simulink model "Scenario_1_fuzzy_tuning"  (R2025b)
settings: Solver=VariableStepAuto  StartTime=0.0  StopTime=10.0  RelTol=1e-3
model workspace (MAT data in the model file):
  Ke = 1
  a = 1
  a1 = 0.1
libraries: fuzblock x2, slpidlib x1
settings Model: Creator=danai  LastModifiedBy=danai

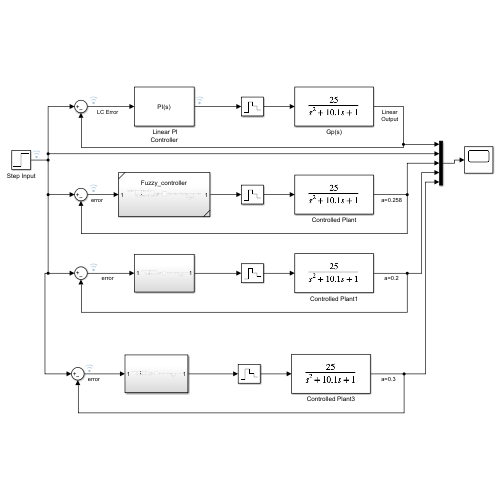
[thumbnail: Simulink's stored preview of the top-level diagram]
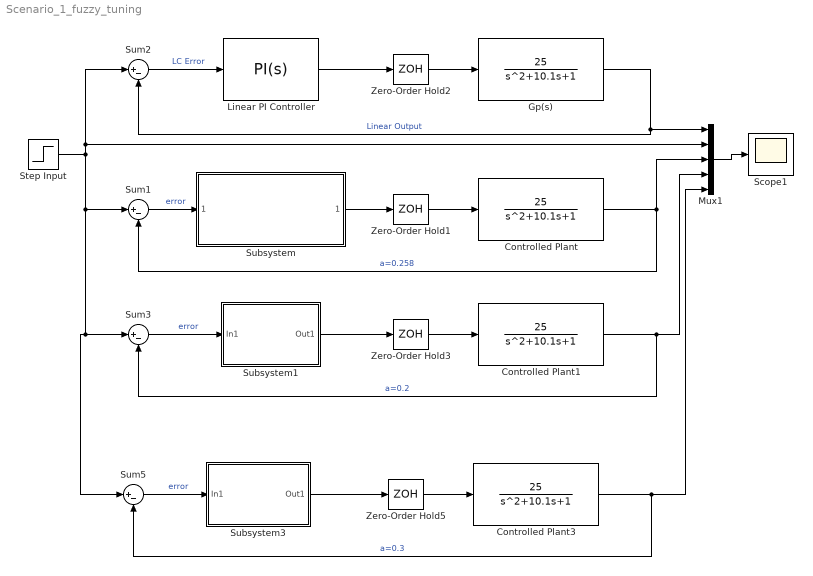
== system Scenario_1_fuzzy_tuning ==
  " Linear PI Controller" : slpidlib/PID Controller  Controller=PI  Form=Parallel  TimeDomain=Continuous-time  UseExternalTs=off  SampleTime=-1  IntegratorMethod=Forward Euler  FilterMethod=Forward Euler  ControllerParametersSource=internal  P=1.34112  I=0.16764  UseKiTs=off  D=0  UseExternalDerivativeSource=off  N=100  UseFilter=on  TunerSelectOption=Transfer Function Based (PID Tuner App)  InitialConditionSource=internal  InitialConditionForIntegrator=0  InitialConditionForFilter=0  DifferentiatorICPrevScaledInput=0  ExternalReset=none  TrackingMode=off  Kt=1  LimitOutput=off  SatLimitsSource=internal  UpperSaturationLimit=inf  LowerSaturationLimit=-inf  LinearizeAsGain=on  AntiWindupMode=none  Kb=1  LimitIntegrator=off  UpperIntegratorSaturationLimit=inf  LowerIntegratorSaturationLimit=-inf  POutMin=[]  POutMax=[]  IOutMin=[]  IOutMax=[]  DOutMin=[]  DOutMax=[]  NOutMin=[]  NOutMax=[]  SumOutMin=[]  SumOutMax=[]  SaturationOutMin=[]  SaturationOutMax=[]  PParamMin=[]  PParamMax=[]  IParamMin=[]  IParamMax=[]  DParamMin=[]  DParamMax=[]  NParamMin=[]  NParamMax=[]  KbParamMin=[]  KbParamMax=[]  KtParamMin=[]  KtParamMax=[]  KbOutMin=[]  KbOutMax=[]  KtOutMin=[]  KtOutMax=[]  IntegratorOutMin=[]  IntegratorOutMax=[]  FilterOutMin=[]  FilterOutMax=[]  SumI1OutMin=[]  SumI1OutMax=[]  SumI2OutMin=[]  SumI2OutMax=[]  SumI3OutMin=[]  SumI3OutMax=[]  SumI4OutMin=[]  SumI4OutMax=[]  SumDOutMin=[]  SumDOutMax=[]  DifferentiatorOutMin=[]  DifferentiatorOutMax=[]  FilterDiffOutCoefMin=[]  FilterDiffOutCoefMax=[]  ReciprocalOutMin=[]  ReciprocalOutMax=[]  SumDenOutMin=[]  SumDenOutMax=[]  SumNumOutMin=[]  SumNumOutMax=[]  DivideOutMin=[]  DivideOutMax=[]  UdiffTsProdOutMin=[]  UdiffTsProdOutMax=[]  NTsProdOutMin=[]  NTsProdOutMax=[]  UintegralTsProdOutMin=[]  UintegralTsProdOutMax=[]  UngainTsProdOutMin=[]  UngainTsProdOutMax=[]  ClampingZeroOutDataTypeStr=Inherit: Inherit via back propagation  ClampingZeroOutMin=[]  ClampingZeroOutMax=[]  FilterDenConstantOutDataTypeStr=Inherit: Inherit via back propagation  FilterDenConstantOutMin=[]  FilterDenConstantOutMax=[]  PCopyOutDataTypeStr=Inherit: Inherit via back propagation  PCopyOutMin=[]  PCopyOutMax=[]  NCopyOutDataTypeStr=Inherit: Inherit via back propagation  NCopyOutMin=[]  NCopyOutMax=[]  IntegratorContinuousStateAttributes=''  IntegratorStateMustResolveToSignalObject=off  IntegratorRTWStateStorageClass=Auto  FilterContinuousStateAttributes=''  FilterStateMustResolveToSignalObject=off  FilterRTWStateStorageClass=Auto  ParallelPVariant=InternalParameters  IdealPVariant=Disabled  IVariant=InternalParameters  DVariant=Disabled  IntegratorVariant=Continuous  SatVariant=Disabled  AWVariant=Passthrough  PCopyVariant=Disabled  TRVariant=Disabled  FdbkBlocksVariant=Forward  IdealPFdbkVariant=Disabled  SatFdbkVariant=Disabled  DerivativeFilterVariant=Disabled  NVariant=Disabled  NCopyVariant=Disabled_SignalSpec  FilterICVariant=Disabled  IntegratorICVariant=InternalICs  ExternalResetVariant=Disabled  TRSumVariant=Passthrough  SumFdbkVariant=Disabled  SumVariant=Sum_PI  TsampFilterVariant=InternalTs  TsampNgainVariant=Passthrough  TsampIntegralVariant=Disabled_SignalSpec  ExternalSaturationOutDataTypeStr=Inherit: Same as second input  DerivativeSourceVariant=Disabled  PreIntVariant=InternalPreInt
  Controlled Plant : TransferFcn  Numerator=[25]  Denominator=[1 10.1 1]
  Controlled Plant1 : TransferFcn  Numerator=[25]  Denominator=[1 10.1 1]
  Controlled Plant3 : TransferFcn  Numerator=[25]  Denominator=[1 10.1 1]
  Gp(s) : TransferFcn  Numerator=[25]  Denominator=[1 10.1 1]
  Mux1 : Mux  Inputs=5
  Scope1 : Scope
      settings: ActiveDisplayYMinimum=-4.7207161874772012  ActiveDisplayYMaximum=84.611232250889316
  Step Input : Step  Before=50  After=50  SampleTime=0.01
  Subsystem : Subsystem  ReferencedSubsystem=Fuzzy_controller
  Subsystem1 : Subsystem
  Subsystem3 : Subsystem
  Sum{1..3,5} (4 alike) : Sum  Inputs=|+-
  Zero-Order Hold{1..3,5} (4 alike) : ZeroOrderHold  SampleTime=-1
  wires:
  Controlled Plant3/1 -> Mux1/5, Sum5/2  "a=0.3"
  Zero-Order Hold2/1 -> Gp(s)/1
  " Linear PI Controller"/1 -> Zero-Order Hold2/1
  Controlled Plant/1 -> Sum1/2, Mux1/3  "a=0.258"
  Zero-Order Hold1/1 -> Controlled Plant/1
  Controlled Plant1/1 -> Mux1/4, Sum3/2  "a=0.2"
  Gp(s)/1 -> Sum2/2, Mux1/1  "Linear Output"
  Sum2/1 -> " Linear PI Controller"/1  "LC Error"
  Zero-Order Hold5/1 -> Controlled Plant3/1
  Step Input/1 -> Sum2/1, Mux1/2, Sum5/1, Sum3/1, Sum1/1
  Mux1/1 -> Scope1/1
  Zero-Order Hold3/1 -> Controlled Plant1/1
  Sum3/1 -> Subsystem1/1(In1)  "error"
  Subsystem1/1(Out1) -> Zero-Order Hold3/1
  Subsystem/1 -> Zero-Order Hold1/1
  Sum1/1 -> Subsystem/1  "error"
  Sum5/1 -> Subsystem3/1(In1)  "error"
  Subsystem3/1(Out1) -> Zero-Order Hold5/1

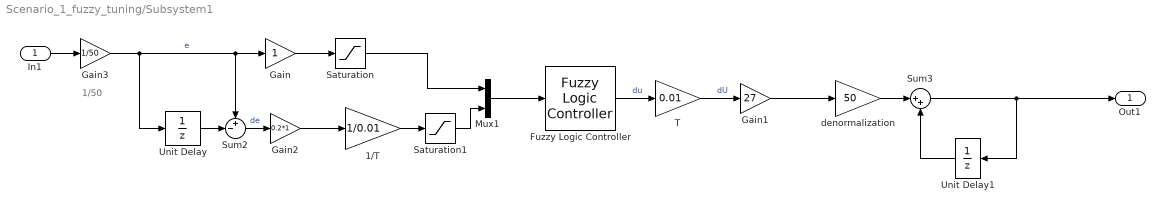
== system Scenario_1_fuzzy_tuning/Subsystem1 ==
  note: 1/50
  In1 : Inport
  1/T : Gain  Gain=1/0.01
  Fuzzy Logic Controller : fuzblock/Fuzzy Logic  Controller  FIS=Trapezi_ergasias_24_MyFIS  OutputSampleNumber=101  DataType=double  UseLookupTable=off  NumBreakpoints=10  FuzzifiedInputs=off  RuleFiringStrengths=off  RuleOutputs=off  AggregatedOutputs=off  SimulateUsing=Interpreted execution  OutOfRangeInputValueMessage=warning  NoRuleFiredMessage=warning  EmptyOutputFuzzySetMessage=warning
  Gain : Gain
  Gain1 : Gain  Gain=27
  Gain2 : Gain  Gain=0.2*1
  Gain3 : Gain  Gain=1/50
  Mux1 : Mux  Inputs=2
  Saturation : Saturate  UpperLimit=1  LowerLimit=-1
  Saturation1 : Saturate  UpperLimit=1  LowerLimit=-1
  Sum2 : Sum  Inputs=+-|
  Sum3 : Sum  Inputs=|++
  T : Gain  Gain=0.01
  Unit Delay : UnitDelay  SampleTime=0.01  HasFrameUpgradeWarning=on
  Unit Delay1 : UnitDelay  SampleTime=0.01  HasFrameUpgradeWarning=on
  denormalization : Gain  Gain=50
  Out1 : Outport
  wires:
  T/1 -> Gain1/1  "dU"
  In1/1 -> Gain3/1
  Sum3/1 -> Out1/1, Unit Delay1/1
  Saturation1/1 -> Mux1/2
  Unit Delay1/1 -> Sum3/2
  Gain3/1 -> Unit Delay/1, Sum2/1, Gain/1  "e"
  Fuzzy Logic Controller/1 -> T/1  "du"
  Unit Delay/1 -> Sum2/2
  Saturation/1 -> Mux1/1
  Gain1/1 -> denormalization/1
  1/T/1 -> Saturation1/1
  Gain/1 -> Saturation/1
  Gain2/1 -> 1/T/1
  Sum2/1 -> Gain2/1  "de"
  Mux1/1 -> Fuzzy Logic Controller/1
  denormalization/1 -> Sum3/1

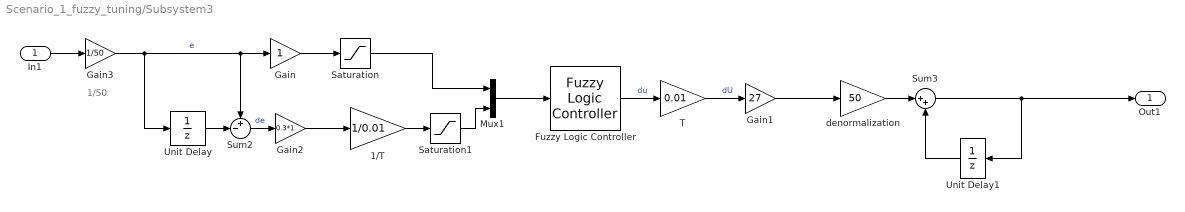
== system Scenario_1_fuzzy_tuning/Subsystem3 ==
  note: 1/50
  In1 : Inport
  1/T : Gain  Gain=1/0.01
  Fuzzy Logic Controller : fuzblock/Fuzzy Logic  Controller  FIS=Trapezi_ergasias_24_MyFIS  OutputSampleNumber=101  DataType=double  UseLookupTable=off  NumBreakpoints=10  FuzzifiedInputs=off  RuleFiringStrengths=off  RuleOutputs=off  AggregatedOutputs=off  SimulateUsing=Interpreted execution  OutOfRangeInputValueMessage=warning  NoRuleFiredMessage=warning  EmptyOutputFuzzySetMessage=warning
  Gain : Gain
  Gain1 : Gain  Gain=27
  Gain2 : Gain  Gain=0.3*1
  Gain3 : Gain  Gain=1/50
  Mux1 : Mux  Inputs=2
  Saturation : Saturate  UpperLimit=1  LowerLimit=-1
  Saturation1 : Saturate  UpperLimit=1  LowerLimit=-1
  Sum2 : Sum  Inputs=+-|
  Sum3 : Sum  Inputs=|++
  T : Gain  Gain=0.01
  Unit Delay : UnitDelay  SampleTime=0.01  HasFrameUpgradeWarning=on
  Unit Delay1 : UnitDelay  SampleTime=0.01  HasFrameUpgradeWarning=on
  denormalization : Gain  Gain=50
  Out1 : Outport
  wires:
  denormalization/1 -> Sum3/1
  1/T/1 -> Saturation1/1
  Saturation/1 -> Mux1/1
  Gain2/1 -> 1/T/1
  Fuzzy Logic Controller/1 -> T/1  "du"
  Unit Delay1/1 -> Sum3/2
  Gain3/1 -> Unit Delay/1, Sum2/1, Gain/1  "e"
  Gain/1 -> Saturation/1
  Gain1/1 -> denormalization/1
  Unit Delay/1 -> Sum2/2
  T/1 -> Gain1/1  "dU"
  Sum2/1 -> Gain2/1  "de"
  Mux1/1 -> Fuzzy Logic Controller/1
  Sum3/1 -> Out1/1, Unit Delay1/1
  Saturation1/1 -> Mux1/2
  In1/1 -> Gain3/1
